simulink model "modelo_completo"  (R2021a)
settings: Solver=VariableStepAuto  StartTime=0.0  StopTime=10.0  RelTol=1e-3
values from neighbouring files (symbols this model uses):
  bah = Meqh*nh*w_posh    (= 720000)    [Data.m]
  bat = Meqt*nt*w_post    (= 675000)    [Data.m]
  beqh = 18.0    (= 18)    [Data.m]
  beqt = bt + (beq_rot*rt^2)/(Rw^2)    (= 27000)    [Data.m]
  bw = 30000.0    (= 30000)    [Data.m]
  cont_mass = max_m    (= 50000)    [Data.m]
  g = 9.80665    [Data.m]    (also in PD_balanceo.m = 9.81)
  Ksah = Meqh*nh*w_posh^2    (= 4318720.37915)    [Data.m]
  Ksat = Meqt*nt*w_post^2    (= 3088564.26247)    [Data.m]
  Ksiah = Meqh*w_posh^3    (= 10361858.7296)    [Data.m]
  Ksiat = Meqt*w_post^3    (= 5652876.56499)    [Data.m]
  Kw = 1800000.0    (= 1800000)    [Data.m]
  Meqh = Mh + (Jmh*rth^2 + Jd)/Rd^2    (= 48014.2222222)    [Data.m]
  Meqt = mt + (Jw+Jm*rt^2)/(Rw^2)    (= 59008)    [Data.m]
  Rd = 0.75    [Data.m]
  rt = 15.0    (= 15)    [Data.m]    (also in main.m = 0)
  rth = 30.0    (= 30)    [Data.m]
  Rw = 0.5    [Data.m]    (also in main.m = 0)
  sp_mass = 15000.0    (= 15000)    [Data.m]
  yt0 = 45.0    (= 45)    [Data.m]
settings Model: Creator=facu_  LastModifiedBy=facu_

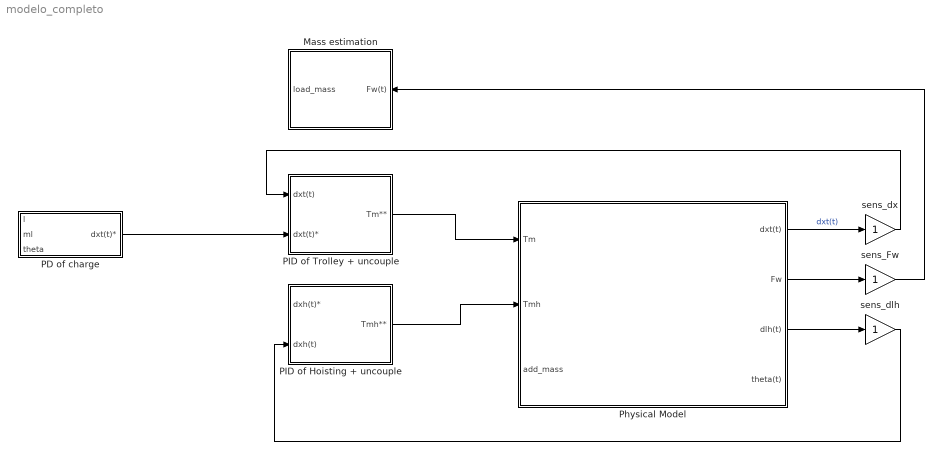
== system modelo_completo ==
  Mass estimation : Subsystem
  "PD of charge " : Subsystem
  "PID of Hoisting + uncouple " : Subsystem
  "PID of Trolley + uncouple " : Subsystem
  Physical Model : Subsystem
  sens_Fw : Gain
  sens_dlh : Gain
  sens_dx : Gain
  wires:
  Physical Model/1(dxt(t)) -> sens_dx/1  "dxt(t)"
  "PID of Trolley + uncouple "/1(Tm**) -> Physical Model/1(Tm)
  "PID of Hoisting + uncouple "/1(Tmh**) -> Physical Model/2(Tmh)
  Physical Model/3(dlh(t)) -> sens_dlh/1
  sens_dx/1 -> "PID of Trolley + uncouple "/1(dxt(t))
  sens_dlh/1 -> "PID of Hoisting + uncouple "/2(dxh(t))
  Physical Model/2(Fw) -> sens_Fw/1
  sens_Fw/1 -> Mass estimation/1(Fw(t))
  "PD of charge "/1(dxt(t)*) -> "PID of Trolley + uncouple "/2(dxt(t)*)

== system modelo_completo/Mass estimation ==
  Fw(t) : Inport
  load_mass : Outport

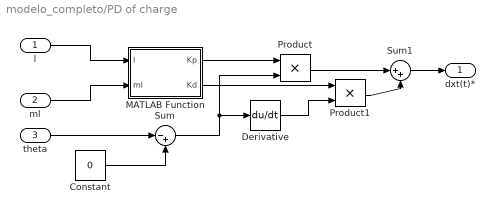
== system modelo_completo/PD of charge  ==
  l : Inport
  ml : Inport  Port=2
  theta : Inport  Port=3
  Constant : Constant  Value=0
  Derivative : Derivative
  MATLAB Function : MATLAB Function  TreatAsAtomicUnit=on
  Product : Product
  Product1 : Product
  Sum : Sum  Inputs=|-+
  Sum1 : Sum  Inputs=|++
  dxt(t)* : Outport
  wires:
  theta/1 -> Sum/1
  Constant/1 -> Sum/2
  l/1 -> MATLAB Function/1(l)
  ml/1 -> MATLAB Function/2(ml)
  Sum/1 -> Product/2, Derivative/1
  Product1/1 -> Sum1/2
  Product/1 -> Sum1/1
  Sum1/1 -> dxt(t)*/1
  MATLAB Function/2(Kd) -> Product1/1
  MATLAB Function/1(Kp) -> Product/1
  Derivative/1 -> Product1/2

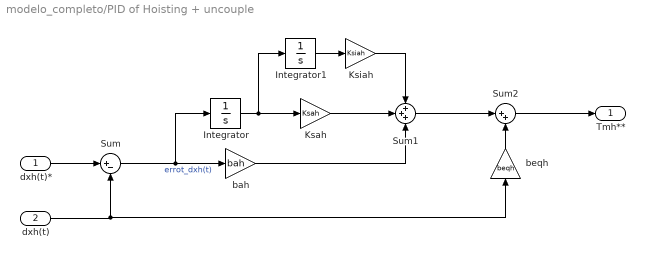
== system modelo_completo/PID of Hoisting + uncouple  ==
  dxh(t)* : Inport
  dxh(t) : Inport  Port=2
  Integrator : Integrator
  Integrator1 : Integrator
  Ksah : Gain  Gain=Ksah
  Ksiah : Gain  Gain=Ksiah
  Sum : Sum  Inputs=|+-
  Sum1 : Sum  Inputs=+++
  Sum2 : Sum  Inputs=|++
  bah : Gain  Gain=bah
  beqh : Gain  Gain=beqh
  Tmh** : Outport
  wires:
  Sum/1 -> bah/1, Integrator/1  "errot_dxh(t)"
  dxh(t)*/1 -> Sum/1
  Sum1/1 -> Sum2/1
  dxh(t)/1 -> beqh/1, Sum/2
  Integrator/1 -> Integrator1/1, Ksah/1
  bah/1 -> Sum1/3
  Ksah/1 -> Sum1/2
  Integrator1/1 -> Ksiah/1
  Ksiah/1 -> Sum1/1
  beqh/1 -> Sum2/2
  Sum2/1 -> Tmh**/1

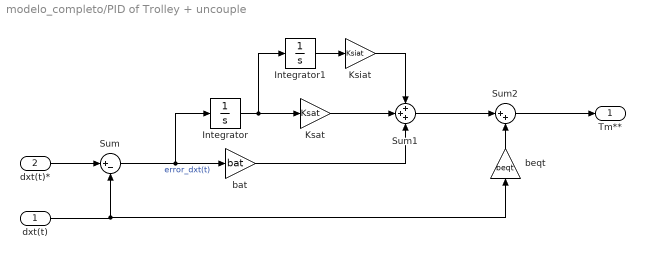
== system modelo_completo/PID of Trolley + uncouple  ==
  dxt(t) : Inport
  dxt(t)* : Inport  Port=2
  Integrator : Integrator
  Integrator1 : Integrator
  Ksat : Gain  Gain=Ksat
  Ksiat : Gain  Gain=Ksiat
  Sum : Sum  Inputs=|+-
  Sum1 : Sum  Inputs=+++
  Sum2 : Sum  Inputs=|++
  bat : Gain  Gain=bat
  beqt : Gain  Gain=beqt
  Tm** : Outport
  wires:
  Sum/1 -> bat/1, Integrator/1  "error_dxt(t)"
  dxt(t)*/1 -> Sum/1
  Sum1/1 -> Sum2/1
  dxt(t)/1 -> beqt/1, Sum/2
  Integrator/1 -> Integrator1/1, Ksat/1
  bat/1 -> Sum1/3
  Ksat/1 -> Sum1/2
  Integrator1/1 -> Ksiat/1
  Ksiat/1 -> Sum1/1
  beqt/1 -> Sum2/2
  Sum2/1 -> Tm**/1

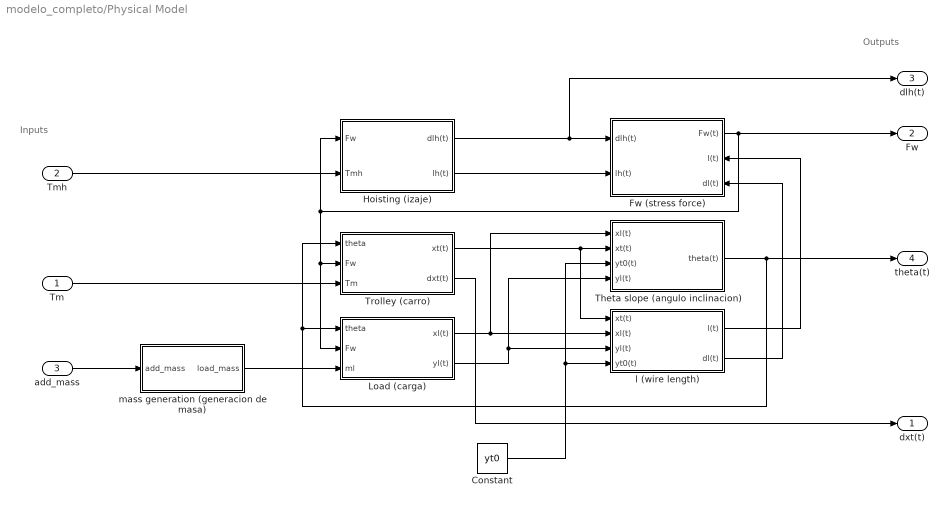
== system modelo_completo/Physical Model ==
  note: Inputs
  note: Outputs
  Tm : Inport
  Tmh : Inport  Port=2
  add_mass : Inport  Port=3
  Constant : Constant  Value=yt0
  Fw (stress force) : Subsystem
      settings: PortSchema="{\"entries\":[{\"content\":{\"sides\":[{\"content\":{\"connectorIds\":[\"In1\",\"In2\"]},\"type\":\"ConnectorPlacement.EquallySpacedRectSide\",\"uuid\":\"ba23d8a5-df88-4a98-9228-1a95ef0572d6\"},{\"content\":{\"connectorIds\":[\"Out1\",\"In3\",\"In4\"],\"side\":\"RIGHT\"},\"type\":\"ConnectorPlacement.EquallySpacedRectSide\",\"uuid\":\"c1b2cc2a-1d19-40da-89ec-405abbf25b58\"},{\"content\":{\"connectorIds\":[],\"side\":\"TOP\"},\"type\":\"ConnectorPlacement.EquallySpacedRectSide\",\"uuid\":\"8c283652-7118-429a-8320-3bc0966db205\"}]},\"type\":\"ConnectorPlacement.EquallySpacedConnector\",\"uuid\":\"7ebc4a5f-6f80-4333-9ee6-9a21b2f2a5d0\"}],\"packageUris\":[\"http://schema.mathworks.com/mf0/Connector/R2020b\"],\"version\":\"1.0\"}"
  Hoisting (izaje) : Subsystem
  Load (carga) : Subsystem
  Theta slope (angulo inclinacion) : Subsystem
  Trolley (carro) : Subsystem
  l (wire length) : Subsystem
  mass generation (generacion de masa) : Subsystem
  dxt(t) : Outport
  Fw : Outport  Port=2
  dlh(t) : Outport  Port=3
  theta(t) : Outport  Port=4
  wires:
  Theta slope (angulo inclinacion)/1(theta(t)) -> theta(t)/1, Load (carga)/1(theta), Trolley (carro)/1(theta)
  Load (carga)/1(xl(t)) -> l (wire length)/2(xl(t)), Theta slope (angulo inclinacion)/1(xl(t))
  Hoisting (izaje)/2(lh(t)) -> Fw (stress force)/2(lh(t))
  Trolley (carro)/1(xt(t)) -> l (wire length)/1(xt(t)), Theta slope (angulo inclinacion)/2(xt(t))
  Fw (stress force)/1(Fw(t)) -> Trolley (carro)/2(Fw), Load (carga)/2(Fw), Hoisting (izaje)/1(Fw), Fw/1
  Constant/1 -> Theta slope (angulo inclinacion)/3(yt0(t)), l (wire length)/4(yt0(t))
  add_mass/1 -> mass generation (generacion de masa)/1(add_mass)
  Load (carga)/2(yl(t)) -> l (wire length)/3(yl(t)), Theta slope (angulo inclinacion)/4(yl(t))
  l (wire length)/1(l(t)) -> Fw (stress force)/3(l(t))
  mass generation (generacion de masa)/1(load_mass) -> Load (carga)/3(ml)
  l (wire length)/2(dl(t)) -> Fw (stress force)/4(dl(t))
  Tmh/1 -> Hoisting (izaje)/2(Tmh)
  Tm/1 -> Trolley (carro)/3(Tm)
  Hoisting (izaje)/1(dlh(t)) -> dlh(t)/1, Fw (stress force)/1(dlh(t))
  Trolley (carro)/2(dxt(t)) -> dxt(t)/1

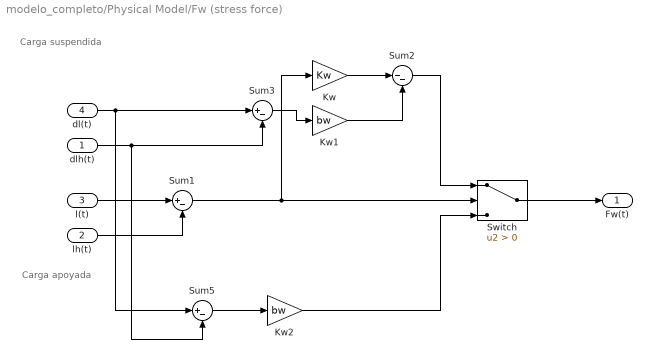
== system modelo_completo/Physical Model/Fw (stress force) ==
  note: Carga suspendida
  note: Carga apoyada
  dlh(t) : Inport
  lh(t) : Inport  Port=2
  l(t) : Inport  Port=3
  dl(t) : Inport  Port=4
  Kw : Gain  Gain=Kw
  Kw1 : Gain  Gain=bw
  Kw2 : Gain  Gain=bw
  Sum1 : Sum  Inputs=|+-
  Sum2 : Sum  Inputs=|--
  Sum3 : Sum  Inputs=|+-
  Sum5 : Sum  Inputs=|+-
  Switch : Switch  Criteria=u2 > Threshold
  Fw(t) : Outport
  wires:
  Switch/1 -> Fw(t)/1
  l(t)/1 -> Sum1/1
  lh(t)/1 -> Sum1/2
  Sum1/1 -> Kw/1, Switch/2
  Sum3/1 -> Kw1/1
  Kw1/1 -> Sum2/2
  Kw/1 -> Sum2/1
  Sum2/1 -> Switch/1
  Sum5/1 -> Kw2/1
  dlh(t)/1 -> Sum5/2, Sum3/2
  dl(t)/1 -> Sum5/1, Sum3/1
  Kw2/1 -> Switch/3

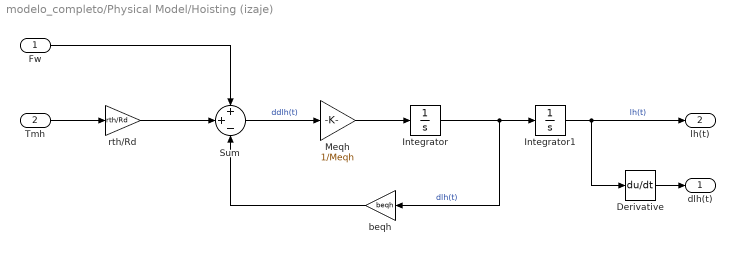
== system modelo_completo/Physical Model/Hoisting (izaje) ==
  Fw : Inport
  Tmh : Inport  Port=2
  Derivative : Derivative
  Integrator : Integrator
  Integrator1 : Integrator
  Meqh : Gain  Gain=1/Meqh
  Sum : Sum  Inputs=++-
  beqh : Gain  Gain=beqh
  rth/Rd : Gain  Gain=rth/Rd
  dlh(t) : Outport
  lh(t) : Outport  Port=2
  wires:
  Fw/1 -> Sum/1
  Tmh/1 -> rth/Rd/1
  rth/Rd/1 -> Sum/2
  Sum/1 -> Meqh/1  "ddlh(t)"
  Meqh/1 -> Integrator/1
  Integrator/1 -> beqh/1, Integrator1/1  "dlh(t)"
  Integrator1/1 -> Derivative/1, lh(t)/1  "lh(t)"
  beqh/1 -> Sum/3
  Derivative/1 -> dlh(t)/1

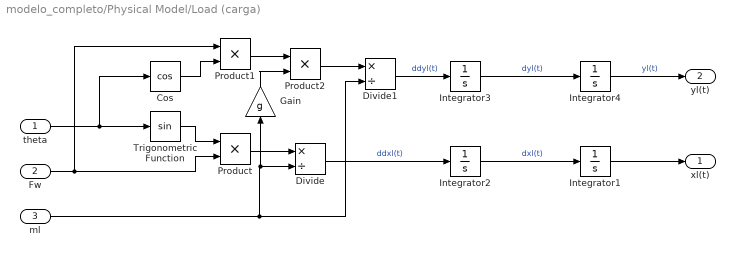
== system modelo_completo/Physical Model/Load (carga) ==
  theta : Inport
  Fw : Inport  Port=2
  ml : Inport  Port=3
  Cos : Trigonometry  Operator=cos
  Divide : Product  Inputs=*/
  Divide1 : Product  Inputs=*/
  Gain : Gain  Gain=g
  Integrator{1..4} (4 alike) : Integrator
  Product : Product
  Product1 : Product
  Product2 : Product
  Trigonometric Function : Trigonometry
  xl(t) : Outport
  yl(t) : Outport  Port=2
  wires:
  theta/1 -> Cos/1, Trigonometric Function/1
  Trigonometric Function/1 -> Product/1
  Fw/1 -> Product1/1, Product/2
  Integrator1/1 -> xl(t)/1
  Integrator2/1 -> Integrator1/1  "dxl(t)"
  ml/1 -> Gain/1, Divide/2, Divide1/2
  Product/1 -> Divide/1
  Divide/1 -> Integrator2/1  "ddxl(t)"
  Cos/1 -> Product1/2
  Product1/1 -> Product2/1
  Gain/1 -> Product2/2
  Product2/1 -> Divide1/1
  Divide1/1 -> Integrator3/1  "ddyl(t)"
  Integrator3/1 -> Integrator4/1  "dyl(t)"
  Integrator4/1 -> yl(t)/1  "yl(t)"

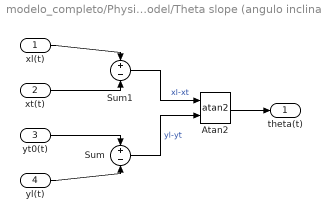
== system modelo_completo/Physical Model/Theta slope (angulo inclinacion) ==
  xl(t) : Inport
  xt(t) : Inport  Port=2
  yt0(t) : Inport  Port=3
  yl(t) : Inport  Port=4
  Atan2 : Trigonometry  Operator=atan2
  Sum : Sum  Inputs=+-
  Sum1 : Sum  Inputs=+-
  theta(t) : Outport
  wires:
  yt0(t)/1 -> Sum/1
  yl(t)/1 -> Sum/2
  xl(t)/1 -> Sum1/1
  xt(t)/1 -> Sum1/2
  Sum1/1 -> Atan2/1  "xl-xt"
  Sum/1 -> Atan2/2  "yl-yt"
  Atan2/1 -> theta(t)/1

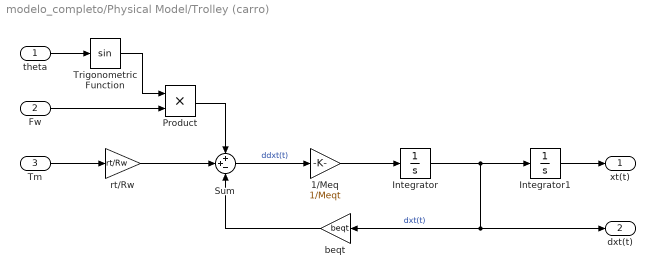
== system modelo_completo/Physical Model/Trolley (carro) ==
  theta : Inport
  Fw : Inport  Port=2
  Tm : Inport  Port=3
  1/Meq : Gain  Gain=1/Meqt
  Integrator : Integrator
  Integrator1 : Integrator
  Product : Product
  Sum : Sum  Inputs=++-
  Trigonometric Function : Trigonometry
  beqt : Gain  Gain=beqt
  rt/Rw : Gain  Gain=rt/Rw
  xt(t) : Outport
  dxt(t) : Outport  Port=2
  wires:
  theta/1 -> Trigonometric Function/1
  Trigonometric Function/1 -> Product/1
  Fw/1 -> Product/2
  Product/1 -> Sum/1
  Tm/1 -> rt/Rw/1
  rt/Rw/1 -> Sum/2
  Sum/1 -> 1/Meq/1  "ddxt(t)"
  1/Meq/1 -> Integrator/1
  Integrator/1 -> Integrator1/1, dxt(t)/1, beqt/1  "dxt(t)"
  Integrator1/1 -> xt(t)/1
  beqt/1 -> Sum/3

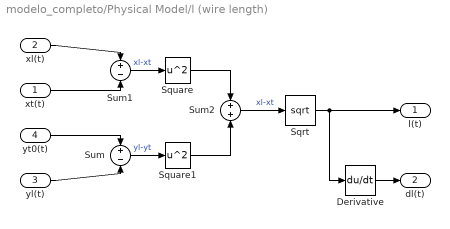
== system modelo_completo/Physical Model/l (wire length) ==
  xt(t) : Inport
  xl(t) : Inport  Port=2
  yl(t) : Inport  Port=3
  yt0(t) : Inport  Port=4
  Derivative : Derivative
  Sqrt : Sqrt  SaturateOnIntegerOverflow=on
  Square : Math  Operator=square  SaturateOnIntegerOverflow=on
  Square1 : Math  Operator=square  SaturateOnIntegerOverflow=on
  Sum : Sum  Inputs=+-
  Sum1 : Sum  Inputs=+-
  Sum2 : Sum
  l(t) : Outport
  dl(t) : Outport  Port=2
  wires:
  yt0(t)/1 -> Sum/1
  yl(t)/1 -> Sum/2
  xl(t)/1 -> Sum1/1
  xt(t)/1 -> Sum1/2
  Sqrt/1 -> Derivative/1, l(t)/1
  Sum1/1 -> Square/1  "xl-xt"
  Sum/1 -> Square1/1  "yl-yt"
  Square/1 -> Sum2/1
  Square1/1 -> Sum2/2
  Sum2/1 -> Sqrt/1  "xl-xt"
  Derivative/1 -> dl(t)/1

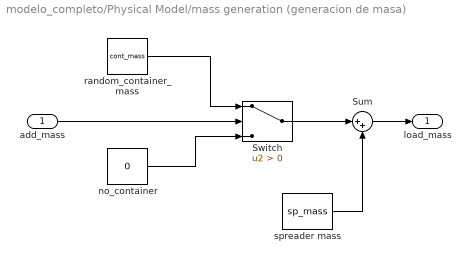
== system modelo_completo/Physical Model/mass generation (generacion de masa) ==
  add_mass : Inport
  Sum : Sum  Inputs=|++
  Switch : Switch  Criteria=u2 > Threshold
  no_container : Constant  Value=0
  random_container_mass : Constant  Value=cont_mass
  spreader mass : Constant  Value=sp_mass
  load_mass : Outport
  wires:
  Sum/1 -> load_mass/1
  spreader mass/1 -> Sum/2
  Switch/1 -> Sum/1
  random_container_mass/1 -> Switch/1
  no_container/1 -> Switch/3
  add_mass/1 -> Switch/2

== matlab function modelo_completo/PD of charge /MATLAB Function ==
  data: l input; Kp output; ml input; Kd output
function [Kp,Kd] = fcn(l, ml)
    wn=800;
    g=9.81;
    Kd = l - ( (Meqt*g)/((wn^2)*(ml+Meqt)) ) ;
    Kp = 2*wn*1*(-l + Kd);
end
